simulink model "Q2_M3"  (R2024b)
settings: Solver=VariableStepAuto  StartTime=0.0  StopTime=100  RelTol=1e-3
model workspace (MAT data in the model file):
  J = 60
  K = 0.5
  L = 1e-06
  R = 0.3
  k = 0.5
settings Model: Creator=chall  LastModifiedBy=chall

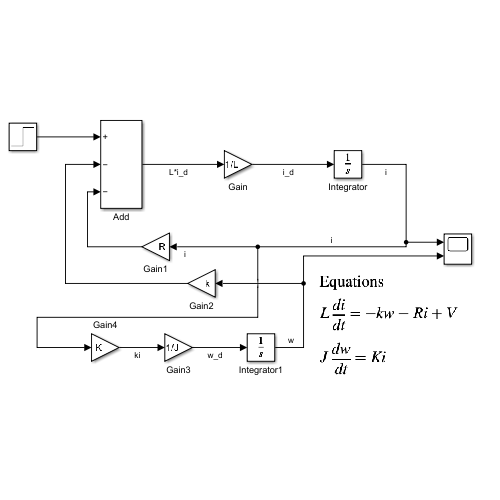
[thumbnail: Simulink's stored preview of the top-level diagram]
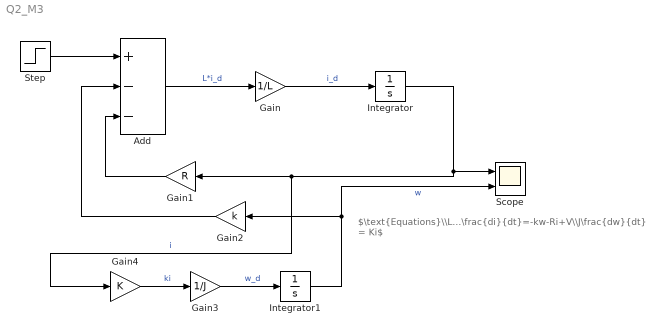
== system Q2_M3 ==
  note: $\text{Equations}\\L\frac{di}{dt}=-kw-Ri+V\\J\frac{dw}{dt} = Ki$
  Add : Sum  Inputs=+--
  Gain : Gain  Gain=1/L
  Gain1 : Gain  Gain=R
  Gain2 : Gain  Gain=k
  Gain3 : Gain  Gain=1/J
  Gain4 : Gain  Gain=K
  Integrator : Integrator
  Integrator1 : Integrator
  Scope : Scope  NumInputPorts=2
  Step : Step  Time=0  SampleTime=0
  wires:
  Add/1 -> Gain/1  "L*i_d"
  Gain/1 -> Integrator/1  "i_d"
  Integrator/1 -> Gain1/1, Gain4/1, Scope/1  "i"
  Gain3/1 -> Integrator1/1  "w_d"
  Integrator1/1 -> Scope/2, Gain2/1  "w"
  Gain1/1 -> Add/3
  Gain2/1 -> Add/2
  Gain4/1 -> Gain3/1  "ki"
  Step/1 -> Add/1
